simulink model "twinBeam_measPosition"  (R2016a)
settings: Solver=FixedStepDiscrete  StartTime=0.0  StopTime=inf  FixedStep=1/10  RelTol=1e-3
InitFcn:
  | load('calibParams.mat')
undefined symbols (not defined in the file or in its folder): IsPositionTracked, IsSkeletonTracked, JointDepthIndices, JointImageIndices, JointTrackingState, JointWorldCoordinates, none, PositionDepthIndices, PositionImageIndices, PositionWorldCoordinates, SegmentationData, SkeletonTrackingID, videoinput
libraries: visiontextngfix x2, imaqlib x1, dspvision x1, visionsinks x1
settings Model: SimulationMode=accelerator  Creator=gurtnmar  LastModifiedBy=marti
settings SolverCC: EnableConcurrentExecution=on
settings DataIOCC: LimitDataPoints=on  SaveFormat=Array  SignalLoggingSaveFormat=ModelDataLogs
settings OptimizationCC: BlockReduction=off  DefaultUnderspecifiedDataType=single  OptimizeBlockIOStorage=off  BufferReuse=off  GlobalBufferReuse=off  ExpressionFolding=off  LocalBlockOutputs=off  EfficientMapNaN2IntZero=off  SimCompilerOptimization=on  AccelVerboseBuild=on
settings DebuggingCC: UnderspecifiedInitializationDetection=Classic  MergeDetectMultiDrivingBlocksExec=none  SolverPrmCheckMsg=warning  MultiTaskDSMMsg=warning  MultiTaskCondExecSysMsg=none  UniqueDataStoreMsg=error  AssertControl=DisableAll  StateNameClashWarn=warning
settings HardwareCC: ProdBitPerPointer=32  ProdLargestAtomicFloat=None  ProdWordSize=32  ProdHWDeviceType=Generic->32-bit x86 compatible  TargetBitPerPointer=64  TargetLongLongMode=on  TargetIntDivRoundTo=Zero  TargetEndianess=LittleEndian  TargetWordSize=64  TargetHWDeviceType=MATLAB Host  ProdEqTarget=off
settings ModelReferenceCC: UpdateModelReferenceTargets=IfOutOfDate  PropagateSignalLabelsOutOfModel=off
settings SFSimCC: SFSimEcho=off
settings RTWCC: Description=Generic Real-Time Target  RTWCompilerOptimization=on
settings CodeAppCC: MaxIdLength=95
settings ConfigComp: CovModelRefEnable=Off  CovSFcnEnable=off

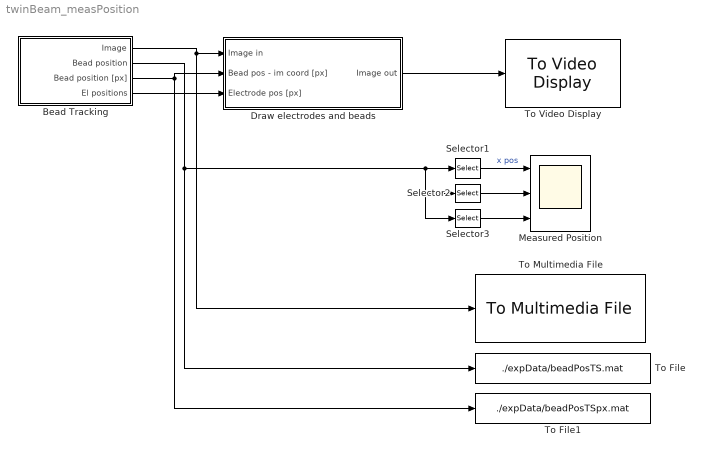
== system twinBeam_measPosition ==
  Bead Tracking : Subsystem  mask{beadSize=55e-6, maxTrackedBeads=1, y_offset=350, calibParamsFile='calibParams.mat', markBeads=on}
      mask prompts: beadSize "Bead size"; maxTrackedBeads "Maximum number of Tracked Beads"; y_offset "Horizontal shift of the image [px]"; calibParamsFile "Calibration parameters file"; markBeads "Mark beads"
  Draw electrodes and beads : Subsystem
  Measured Position : Scope  NumInputPorts=3
  Selector1 : Selector  NumberOfDimensions=2  IndexMode=Zero-based  InputPortWidth=3  IndexOptions=Select all,Index vector (dialog)  Indices=[1 3],0  OutputSizes=1,1
  Selector2 : Selector  NumberOfDimensions=2  IndexMode=Zero-based  InputPortWidth=3  IndexOptions=Select all,Index vector (dialog)  Indices=[1 3],0  OutputSizes=1,1
  Selector3 : Selector  NumberOfDimensions=2  IndexMode=Zero-based  InputPortWidth=3  IndexOptions=Select all,Index vector (dialog)  Indices=[1 3],0  OutputSizes=1,1
  To File : ToFile  Filename=./expData/beadPosTS.mat  MatrixName=beadPos  SaveFormat=Timeseries
  To File1 : ToFile  Filename=./expData/beadPosTSpx.mat  MatrixName=beadPos  SaveFormat=Timeseries
  To Multimedia File : dspvision/To Multimedia File  outputFilename=./expData/output.avi  streamSelection=Video only  videoCompressor=None (uncompressed)  audioCompressor=None (uncompressed)  imagePorts=One multidimensional signal  fileType=AVI  audioDatatype=Determine from input data type  fourcc=RGB  videoQuality=75  mj2000CompFactor=10
  To Video Display : visionsinks/To Video Display  windowSizeMode=True size (1:1)  openAtMdlStart=on  fullScreen=off  videoWindowX=-1181  videoWindowY=-201  saveWindowSize=off  videoWindowWidth=256  videoWindowHeight=256  inputColorFormat=RGB  inputType=Obsolete  imagePorts=One multidimensional signal  OutputDevice=On-screen video monitor  dataOrg=Column-major  isWindowOpen=on
  wires:
  Bead Tracking/2(Bead position) -> To File/1, Selector1/1, Selector3/1, Selector2/1
  Bead Tracking/1(Image) -> Draw electrodes and beads/1(Image in), To Multimedia File/1
  Bead Tracking/3(Bead position [px]) -> Draw electrodes and beads/2(Bead pos - im coord [px]), To File1/1
  Bead Tracking/4(El positions) -> Draw electrodes and beads/3(Electrode pos [px])
  Draw electrodes and beads/1(Image out) -> To Video Display/1
  Selector3/1 -> Measured Position/3
  Selector2/1 -> Measured Position/2
  Selector1/1 -> Measured Position/1  "x pos"

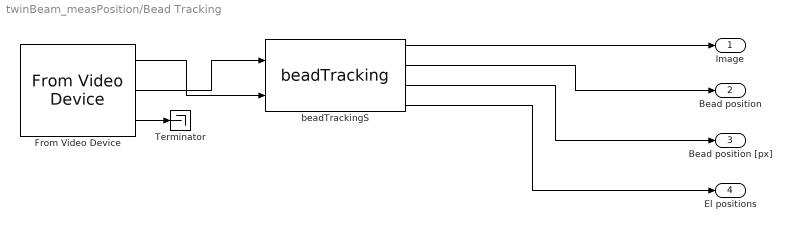
== system twinBeam_measPosition/Bead Tracking ==
  From Video Device : imaqlib/From Video Device  DeviceMenu=(none)  Device=winvideo 1 (e-con s 1MP Bayer RGB Camera)  ObjConstructor=videoinput('winvideo', 1)  VideoFormatMenu=(none)  VideoFormat=BY8 _1280x960  VideoSource=input1  ROIPosition=[0 350 960 512]  EnableHWTrigger=off  TriggerConfiguration=none/none  SampleTime=1/10  OutputPortsMode=Separate color signals  DataType=single  CanDoHWTrigger=no  ReturnedColorSpace=bayer  BlockHandle=1913.0001  ROIWidth=512  ROIHeight=960  ROIColumn=350  ROIRow=0  EngXMLPath=C:\Program Files\MATLAB\R2016a\toolbox\imaq\imaq\private  DevXMLPath=C:\Program Files\MATLAB\R2016a\toolbox\imaq\imaqadaptors\win64  EngLibPath=C:\Program Files\MATLAB\R2016a\toolbox\imaq\imaqblks\imaqmex\win64  ColorSpace=bayer  BayerSensorAlignment=grbg  AllMetadata=IsPositionTracked;IsSkeletonTracked;JointDepthIndices;JointImageIndices;JointTrackingState;JointWorldCoordinates;PositionDepthIndices;PositionImageIndices;PositionWorldCoordinates;SegmentationData;SkeletonTrackingID
  Terminator : Terminator
  beadTrackingS : M-S-Function  FunctionName=beadTracking  Parameters=beadSize,maxTrackedBeads,y_offset,markBeads,calibParamsFile
  Image : Outport
  Bead position : Outport  Port=2
  Bead position [px] : Outport  Port=3
  El positions : Outport  Port=4
  wires:
  beadTrackingS/1 -> Image/1
  From Video Device/1 -> beadTrackingS/2
  From Video Device/3 -> Terminator/1
  From Video Device/2 -> beadTrackingS/1
  beadTrackingS/2 -> Bead position/1
  beadTrackingS/3 -> Bead position [px]/1
  beadTrackingS/4 -> El positions/1

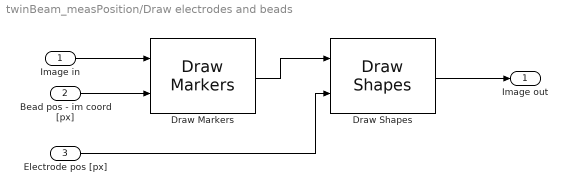
== system twinBeam_measPosition/Draw electrodes and beads ==
  Image in : Inport
  Bead pos - im coord [px] : Inport  Port=2
  Electrode pos [px] : Inport  Port=3
  Draw Markers : visiontextngfix/Draw Markers  shape=X-mark  size=2  fill=off  fillClrSource=Specify via dialog  display=White  intensity=200  color=[255 255 0]  opacity=0.6  viewport=Entire image  antialiasing=off  inType=Obsolete  imagePorts=One multidimensional signal  prodOutputMode=Binary point scaling  prodOutputWordLength=32  prodOutputFracLength=14  memoryMode=Specify word length  memoryWordLength=16  memoryFracLength=15  roundingMode=Floor  overflowMode=off
  Draw Shapes : visiontextngfix/Draw Shapes  shape=Lines  fill=off  lineWidth=1  fillClrSource=Specify via dialog  display=Black  intensity=200  color=[200 255 100]  opacity=0.6  viewport=Entire image  antialiasing=off  inType=Obsolete  imagePorts=One multidimensional signal  prodOutputMode=Binary point scaling  prodOutputWordLength=32  prodOutputFracLength=14  memoryMode=Specify word length  memoryWordLength=16  memoryFracLength=15  roundingMode=Floor  overflowMode=off
  Image out : Outport
  wires:
  Image in/1 -> Draw Markers/1
  Bead pos - im coord [px]/1 -> Draw Markers/2
  Electrode pos [px]/1 -> Draw Shapes/2
  Draw Markers/1 -> Draw Shapes/1
  Draw Shapes/1 -> Image out/1
